simulink model "LPV_mimo_ex_mdl"  (R2016a)
settings: Solver=VariableStepAuto  StartTime=0.0  StopTime=100  RelTol=1e-3
values from neighbouring files (symbols this model uses):
  A0 = [0 1; -0.3  -0.6]    [LPV_mimo_ex.m]
  A1 = [0 0;  0    -0.6]    [LPV_mimo_ex.m]
  A2 = [0 0; -0.01  0]    [LPV_mimo_ex.m]
  B = eye(2)    [LPV_mimo_ex.m]
  C = eye(2)    [LPV_mimo_ex.m]
  Delta = usample(ultidyn('Delta',[no ni]))    [LPV_mimo_ex.m]    (also in LTI_mimo_ex.m; LTI_siso_ex.m)
  Ts = 1    [LPV_mimo_ex.m]    (also in LTI_mimo_ex.m = 0.01; LTI_siso_ex.m = 0.01)
libraries: cstblocks x4, slident x1
settings Model: Creator=fbianchi  LastModifiedBy=fbianchi

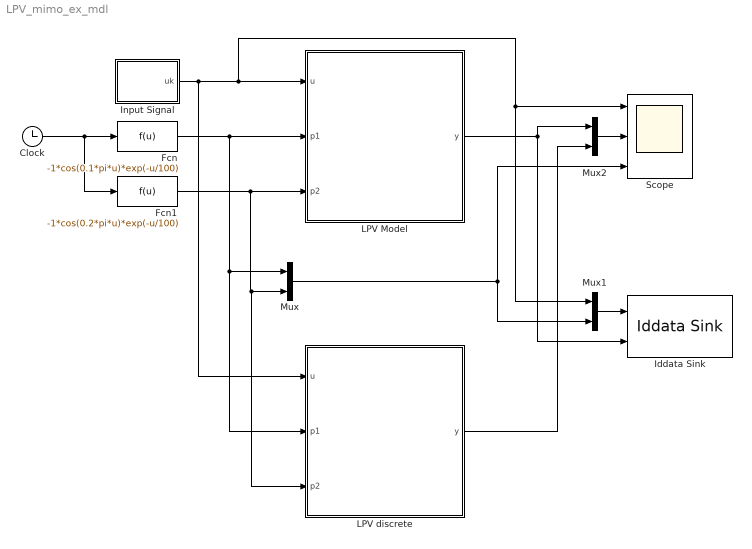
== system LPV_mimo_ex_mdl ==
  Clock : Clock
  Fcn : Fcn  Expr=-1*cos(0.1*pi*u)*exp(-u/100)
  Fcn1 : Fcn  Expr=-1*cos(0.2*pi*u)*exp(-u/100)
  Iddata Sink : slident/Iddata Sink  datasetname=data  Ts=Ts  isu=on  isy=on
  Input Signal : Subsystem
  LPV Model : Subsystem
  LPV discrete : Subsystem
  Mux : Mux  Inputs=2
  Mux1 : Mux  Inputs=[2 2]
  Mux2 : Mux  Inputs=[2 2]
  Scope : Scope  NumInputPorts=3
  wires:
  Clock/1 -> Fcn1/1, Fcn/1
  Fcn/1 -> LPV discrete/2(p1), Mux/1, LPV Model/2(p1)
  Fcn1/1 -> LPV discrete/3(p2), Mux/2, LPV Model/3(p2)
  Input Signal/1(uk) -> LPV discrete/1(u), Mux1/1, Scope/1, LPV Model/1(u)
  LPV Model/1(y) -> Mux2/1, Iddata Sink/2
  Mux/1 -> Mux1/2, Scope/3
  Mux1/1 -> Iddata Sink/1
  Mux2/1 -> Scope/2
  LPV discrete/1(y) -> Mux2/2

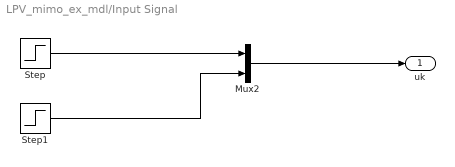
== system LPV_mimo_ex_mdl/Input Signal ==
  Mux2 : Mux  Inputs=2
  Step : Step  Time=30  SampleTime=0
  Step1 : Step  Time=10  SampleTime=0
  uk : Outport
  wires:
  Step1/1 -> Mux2/2
  Mux2/1 -> uk/1
  Step/1 -> Mux2/1

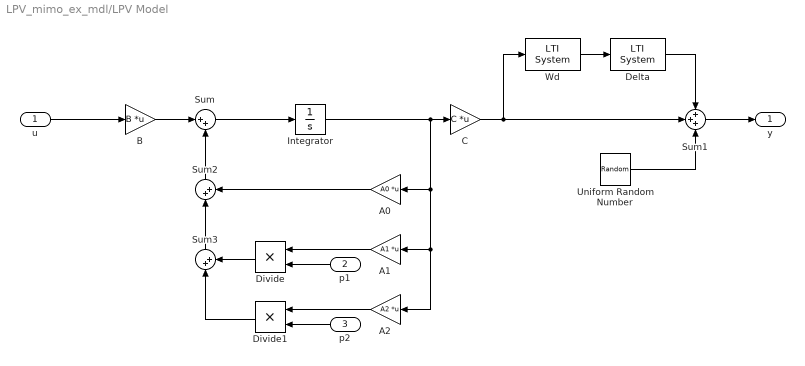
== system LPV_mimo_ex_mdl/LPV Model ==
  u : Inport
  p1 : Inport  Port=2
  p2 : Inport  Port=3
  A0 : Gain  Gain=A0  Multiplication=Matrix(K*u)
  A1 : Gain  Gain=A1  Multiplication=Matrix(K*u)
  A2 : Gain  Gain=A2  Multiplication=Matrix(K*u)
  B : Gain  Gain=B  Multiplication=Matrix(K*u)
  C : Gain  Gain=C  Multiplication=Matrix(K*u)
  Delta : cstblocks/LTI System  sys=Delta  IC=[]
  Divide : Product  Inputs=**
  Divide1 : Product  Inputs=**
  Integrator : Integrator
  Sum : Sum  Inputs=|++
  Sum1 : Sum  Inputs=+++
  Sum2 : Sum  Inputs=|++
  Sum3 : Sum  Inputs=|++
  Uniform Random Number : UniformRandomNumber  Minimum=-0.1  Maximum=0.1  SampleTime=Ts
  Wd : cstblocks/LTI System  sys=Wdc  IC=[]
  y : Outport
  wires:
  p1/1 -> Divide/2
  B/1 -> Sum/1
  u/1 -> B/1
  p2/1 -> Divide1/2
  A1/1 -> Divide/1
  Sum3/1 -> Sum2/1
  Sum2/1 -> Sum/2
  Sum/1 -> Integrator/1
  Divide/1 -> Sum3/2
  Divide1/1 -> Sum3/1
  A2/1 -> Divide1/1
  Integrator/1 -> C/1, A1/1, A2/1, A0/1
  A0/1 -> Sum2/2
  Wd/1 -> Delta/1
  C/1 -> Sum1/2, Wd/1
  Delta/1 -> Sum1/1
  Sum1/1 -> y/1
  Uniform Random Number/1 -> Sum1/3

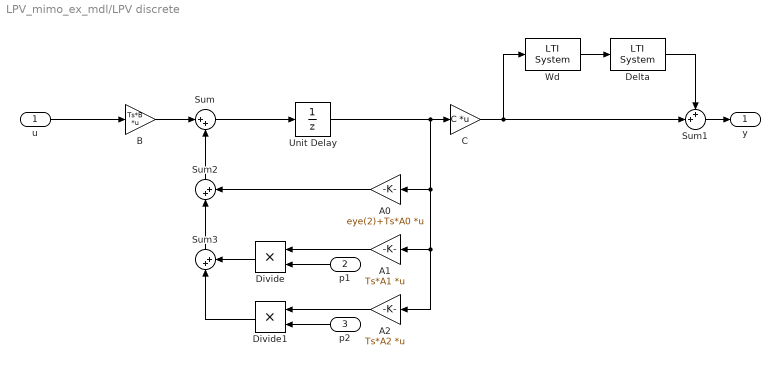
== system LPV_mimo_ex_mdl/LPV discrete ==
  u : Inport
  p1 : Inport  Port=2
  p2 : Inport  Port=3
  A0 : Gain  Gain=eye(2)+Ts*A0  Multiplication=Matrix(K*u)
  A1 : Gain  Gain=Ts*A1  Multiplication=Matrix(K*u)
  A2 : Gain  Gain=Ts*A2  Multiplication=Matrix(K*u)
  B : Gain  Gain=Ts*B  Multiplication=Matrix(K*u)
  C : Gain  Gain=C  Multiplication=Matrix(K*u)
  Delta : cstblocks/LTI System  sys=c2d(Delta,Ts)  IC=[]
  Divide : Product  Inputs=**
  Divide1 : Product  Inputs=**
  Sum : Sum  Inputs=|++
  Sum1 : Sum  Inputs=++|
  Sum2 : Sum  Inputs=|++
  Sum3 : Sum  Inputs=|++
  Unit Delay : UnitDelay  SampleTime=Ts
  Wd : cstblocks/LTI System  sys=Wd  IC=[]
  y : Outport
  wires:
  A0/1 -> Sum2/2
  Unit Delay/1 -> A0/1, A2/1, A1/1, C/1
  A2/1 -> Divide1/1
  Divide1/1 -> Sum3/1
  Divide/1 -> Sum3/2
  Sum/1 -> Unit Delay/1
  Sum2/1 -> Sum/2
  Sum3/1 -> Sum2/1
  A1/1 -> Divide/1
  p2/1 -> Divide1/2
  u/1 -> B/1
  B/1 -> Sum/1
  p1/1 -> Divide/2
  Wd/1 -> Delta/1
  C/1 -> Sum1/2, Wd/1
  Delta/1 -> Sum1/1
  Sum1/1 -> y/1
